simulink model "Y_DFK_MDL_SV"  (R2013a)
settings: Solver=ode45  StartTime=0.0  StopTime=inf  RelTol=1e-3
undefined symbols (not defined in the file or in its folder): ToSimulink_Y_Signals2VRML, Y_DFK_SV, Y_Ja_SV, Y_Jg_SV
libraries: simulink x6, vrlib x1
settings Model: Creator=Angel  LastModifiedBy=root

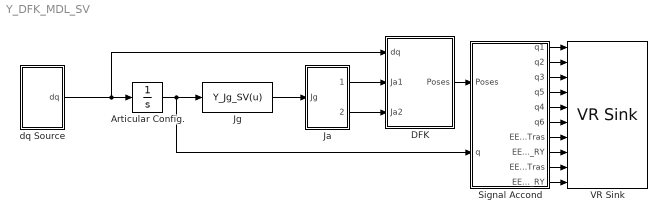
== system Y_DFK_MDL_SV ==
  Articular Config. : Integrator
  DFK : Subsystem
  Ja : Subsystem
  Jg : MATLABFcn  MATLABFcn=Y_Jg_SV(u)  OutputDimensions=42
  Signal Accond : Subsystem
  VR Sink : vrlib/VR Sink  InstantiateOnLoad=on  SampleTime=0.1  ViewEnable=on  RemoteChange=off  RemoteView=off  FieldsWritten=Q_1.rotation.4.1.1.double#Q_2.rotation.4.1.1.double#Q_3_Der.rotation.4.1.1.double#Q_5.rotation.4.1.1.double#Q_4_Izq.rotation.4.1.1.double#Q_6.rotation.4.1.1.double#Tras_Objective1.translation.3.1.1.double#RY_Obj1.rotation.4.1.1.double#Tras_Objective2.translation.3.1.1.double#RY_Obj2.rotation.4.1.1.double  WorldFileName=Y.WRL  AutoView=off  VideoDimensions=[]  AllowVariableSize=off
  dq Source : Subsystem
  wires:
  dq Source/1(dq) -> DFK/1(dq), Articular Config./1
  Articular Config./1 -> Signal Accond/2(q), Jg/1
  Jg/1 -> Ja/1(Jg)
  Ja/1(Jan1) -> DFK/2(Ja1)
  Ja/2(Jan2) -> DFK/3(Ja2)
  DFK/1(Poses) -> Signal Accond/1(Poses)
  Signal Accond/5(q4) -> VR Sink/5
  Signal Accond/1(q1) -> VR Sink/1
  Signal Accond/2(q2) -> VR Sink/2
  Signal Accond/3(q3) -> VR Sink/3
  Signal Accond/4(q5) -> VR Sink/4
  Signal Accond/6(q6) -> VR Sink/6
  Signal Accond/7(EE_Der_Tras) -> VR Sink/7
  Signal Accond/9(EE_Izq_Tras) -> VR Sink/9
  Signal Accond/8(EE_Der_RY) -> VR Sink/8
  Signal Accond/10(EE_Izq_RY) -> VR Sink/10

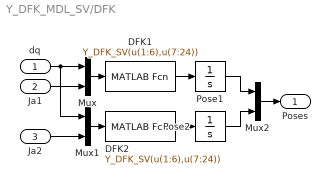
== system Y_DFK_MDL_SV/DFK ==
  dq : Inport
  Ja1 : Inport  Port=2
  Ja2 : Inport  Port=3
  DFK1 : MATLABFcn  MATLABFcn=Y_DFK_SV(u(1:6),u(7:24))  OutputDimensions=3
  DFK2 : MATLABFcn  MATLABFcn=Y_DFK_SV(u(1:6),u(7:24))  OutputDimensions=3
  Mux : Mux  Inputs=2
  Mux1 : Mux  Inputs=2
  Mux2 : Mux  Inputs=2
  Pose1 : Integrator  InitialCondition=[2.8284;6.8284;0]
  Pose2 : Integrator  InitialCondition=[-2.8284;6.8284;0]
  Poses : Outport
  wires:
  DFK1/1 -> Pose1/1
  dq/1 -> Mux/1, Mux1/1
  Mux2/1 -> Poses/1
  Pose2/1 -> Mux2/2
  Ja2/1 -> Mux1/2
  Ja1/1 -> Mux/2
  Mux/1 -> DFK1/1
  Mux1/1 -> DFK2/1
  Pose1/1 -> Mux2/1
  DFK2/1 -> Pose2/1

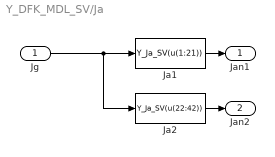
== system Y_DFK_MDL_SV/Ja ==
  Jg : Inport
  Ja1 : MATLABFcn  MATLABFcn=Y_Ja_SV(u(1:21))  OutputDimensions=18
  Ja2 : MATLABFcn  MATLABFcn=Y_Ja_SV(u(22:42))  OutputDimensions=18
  Jan1 : Outport
  Jan2 : Outport  Port=2
  wires:
  Jg/1 -> Ja2/1, Ja1/1
  Ja2/1 -> Jan2/1
  Ja1/1 -> Jan1/1

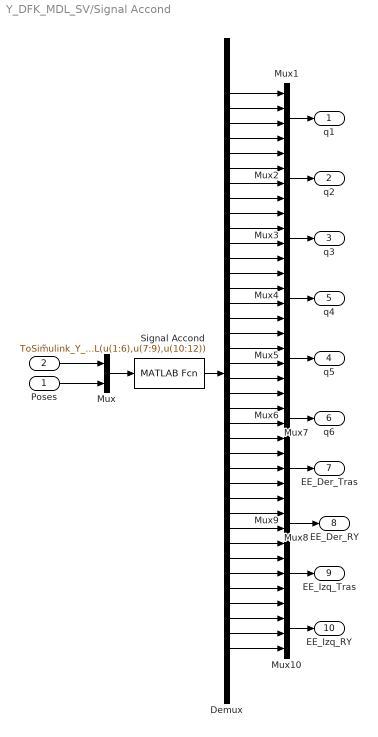
== system Y_DFK_MDL_SV/Signal Accond ==
  Poses : Inport
  q : Inport  Port=2
  Demux : Demux  Outputs=38
  Mux : Mux  Inputs=2
  Mux{1..6,9..10} (8 alike) : Mux
  Mux7 : Mux  Inputs=3
  Mux8 : Mux  Inputs=3
  Signal Accond : MATLABFcn  MATLABFcn=ToSimulink_Y_Signals2VRML(u(1:6),u(7:9),u(10:12))  OutputDimensions=38
  q1 : Outport
  q2 : Outport  Port=2
  q3 : Outport  Port=3
  q5 : Outport  Port=4
  q4 : Outport  Port=5
  q6 : Outport  Port=6
  EE_Der_Tras : Outport  Port=7
  EE_Der_RY : Outport  Port=8
  EE_Izq_Tras : Outport  Port=9
  EE_Izq_RY : Outport  Port=10
  wires:
  q/1 -> Mux/1
  Poses/1 -> Mux/2
  Mux/1 -> Signal Accond/1
  Signal Accond/1 -> Demux/1
  Mux1/1 -> q1/1
  Mux2/1 -> q2/1
  Mux3/1 -> q3/1
  Mux4/1 -> q4/1
  Mux5/1 -> q5/1
  Mux6/1 -> q6/1
  Mux7/1 -> EE_Der_Tras/1
  Mux8/1 -> EE_Izq_Tras/1
  Mux10/1 -> EE_Izq_RY/1
  Mux9/1 -> EE_Der_RY/1
  Demux/32 -> Mux8/1
  Demux/9 -> Mux3/1
  Demux/10 -> Mux3/2
  Demux/18 -> Mux5/2
  Demux/37 -> Mux10/3
  Demux/34 -> Mux8/3
  Demux/19 -> Mux5/3
  Demux/17 -> Mux5/1
  Demux/38 -> Mux10/4
  Demux/5 -> Mux2/1
  Demux/16 -> Mux4/4
  Demux/30 -> Mux9/3
  Demux/11 -> Mux3/3
  Demux/21 -> Mux6/1
  Demux/7 -> Mux2/3
  Demux/29 -> Mux9/2
  Demux/23 -> Mux6/3
  Demux/27 -> Mux7/3
  Demux/6 -> Mux2/2
  Demux/26 -> Mux7/2
  Demux/24 -> Mux6/4
  Demux/15 -> Mux4/3
  Demux/22 -> Mux6/2
  Demux/31 -> Mux9/4
  Demux/33 -> Mux8/2
  Demux/36 -> Mux10/2
  Demux/25 -> Mux7/1
  Demux/13 -> Mux4/1
  Demux/4 -> Mux1/4
  Demux/1 -> Mux1/1
  Demux/2 -> Mux1/2
  Demux/12 -> Mux3/4
  Demux/8 -> Mux2/4
  Demux/35 -> Mux10/1
  Demux/3 -> Mux1/3
  Demux/20 -> Mux5/4
  Demux/14 -> Mux4/2
  Demux/28 -> Mux9/1

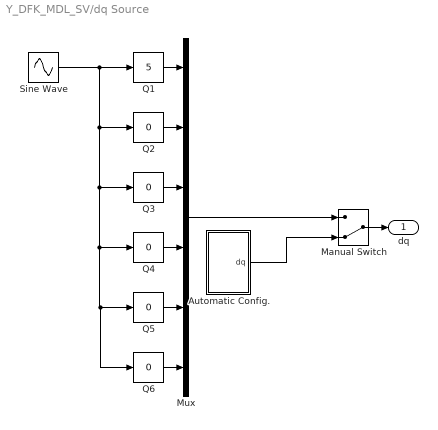
== system Y_DFK_MDL_SV/dq Source ==
  Automatic Config. : Subsystem
  Manual Switch : ManualSwitch  CurrentSetting=0
  Mux : Mux  Inputs=6
  Q1 : simulink/Math Operations/Slider Gain  low=-0.6  gain=5  high=5
  Q{2..6} (5 alike) : simulink/Math Operations/Slider Gain  low=-0.6  gain=0  high=0.6
  Sine Wave : Sin  SampleTime=0
  dq : Outport
  wires:
  Mux/1 -> Manual Switch/1
  Automatic Config./1(dq) -> Manual Switch/2
  Q1/1 -> Mux/1
  Q5/1 -> Mux/5
  Q6/1 -> Mux/6
  Q4/1 -> Mux/4
  Q3/1 -> Mux/3
  Q2/1 -> Mux/2
  Sine Wave/1 -> Q6/1, Q5/1, Q4/1, Q3/1, Q2/1, Q1/1
  Manual Switch/1 -> dq/1

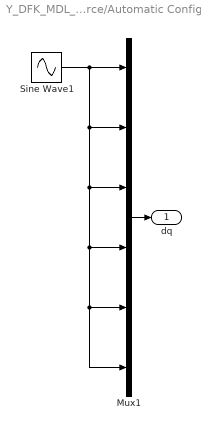
== system Y_DFK_MDL_SV/dq Source/Automatic Config. ==
  Mux1 : Mux  Inputs=6
  Sine Wave1 : Sin  Amplitude=0.5  SampleTime=0
  dq : Outport
  wires:
  Sine Wave1/1 -> Mux1/6, Mux1/5, Mux1/4, Mux1/3, Mux1/2, Mux1/1
  Mux1/1 -> dq/1
